simulink model "VHF_central_unit"  (R2024a)
settings: Solver=FixedStepDiscrete  StartTime=0.0  StopTime=10.0  FixedStep=0.001  RelTol=1e-3  EnableMultiTasking=on
PreLoadFcn:
  | try
  | MDL_install;
  | catch
  | end
InitFcn:
  | EcoCoder_PreCheckLic();
undefined symbols (not defined in the file or in its folder): C_ROTSPD_ZERO, C_SOC_ZERO, h, km, s, V
libraries: CoderSF_BSW_Libs x222, SF_CanService_Libs x16, CoderSF_ADC2Volt_Libs x6, CoderSF_6AxisMEMS_Libs x6, canmsglib x3, EV_ASWLibs x2, simulink x2, Chassis_stability_controllers x1, CoderSF_KeyCycle_Libs x1
(part 1 of 4)
CloseFcn:
  | try
  | MDL_uninstall;
  | catch
  | end
settings Model: Param_HCUVersion=EV22297A  Creator=HXL  LastModifiedBy=Henrique Mesquita
settings SolverCC: AlgebraicLoopSolver=TrustRegion
settings DataIOCC: ExternalInput=InputData  SaveFormat=Structure  SignalLoggingSaveFormat=ModelDataLogs  SaveOutput=off  SignalLogging=off  DSMLogging=off  SaveTime=off  ReturnWorkspaceOutputs=off
settings OptimizationCC: DefaultParameterBehavior=Inlined  InlineInvariantSignals=on  EnhancedBackFolding=on  StrengthReduction=on  EnableMemcpy=off  PassReuseOutputArgsAs=Individual arguments  ExpressionDepthLimit=2147483647  EfficientFloat2IntCast=on  LifeSpan=1  SimCompilerOptimization=on  OptimizeBlockOrder=speed  DifferentSizesBufferReuse=on  EfficientTunableParamExpr=on
settings DebuggingCC: AlgebraicLoopMsg=none  ArtificialAlgebraicLoopMsg=none  SaveWithDisabledLinksMsg=none  SaveWithParameterizedLinksMsg=none  CheckSSInitialOutputMsg=off  UnderspecifiedInitializationDetection=Classic  MergeDetectMultiDrivingBlocksExec=none  SignalResolutionControl=TryResolveAll  BlockPriorityViolationMsg=error  MinStepSizeMsg=none  InheritedTsInSrcMsg=none  MultiTaskDSMMsg=none  MultiTaskCondExecSysMsg=none  MultiTaskRateTransMsg=warning  TasksWithSamePriorityMsg=none  SigSpecEnsureSampleTimeMsg=none  IntegerOverflowMsg=error  Int32ToFloatConvMsg=none  ParameterPrecisionLossMsg=none  ParameterTunabilityLossMsg=none  FixptConstOverflowMsg=error  FcnCallInpInsideContextMsg=warning  UnconnectedInputMsg=error  UnconnectedOutputMsg=error  UnconnectedLineMsg=error  FrameProcessingCompatibilityMsg=none  BusObjectLabelMismatch=none  RootOutportRequireBusObject=none  UnknownTsInhSupMsg=none  ModelReferenceDataLoggingMessage=none  OperatingPointInterfaceChecksumMismatchMsg=none  SFUnusedDataAndEventsDiag=none  SFUnexpectedBacktrackingDiag=none  SFInvalidInputDataAccessInChartInitDiag=none  SFNoUnconditionalDefaultTransitionDiag=none  SFTransitionOutsideNaturalParentDiag=none  SFUnreachableExecutionPathDiag=none  SFExecutionAtInitializationDiag=none  IntegerSaturationMsg=error  ArithmeticOperatorsInVariantConditions=warning
settings HardwareCC: ProdBitPerPointer=32  ProdBitPerSizeT=32  ProdBitPerPtrDiffT=32  ProdLargestAtomicFloat=None  ProdWordSize=32  ProdHWDeviceType=Infineon->TriCore  TargetIntDivRoundTo=Zero  TargetEndianess=BigEndian  TargetHWDeviceType=Freescale->MPC55xx
settings ModelReferenceCC: UpdateModelReferenceTargets=Force  ModelReferenceNumInstancesAllowed=Single  PropagateSignalLabelsOutOfModel=off
settings SFSimCC: SFSimEcho=off  SimUseLocalCustomCode=off  MATLABDynamicMemAlloc=off  CustomCodeUndefinedFunction=UseInterfaceOnly
settings RTWCC: Description=Ecotrons TC2xx  SystemTargetFile=EcoCoderTC27x.tlc  GenerateMakefile=off  TemplateMakefile=ert_default_tmf  RTWVerbose=off  RetainRTWFile=on  RTWUseLocalCustomCode=off  RTWCompilerOptimization=on  GPUComputeCapability=3.5
settings CodeAppCC: IgnoreCustomStorageClasses=off  OperatorAnnotations=on  CustomSymbolStrGlobalVar=$N$M  CustomSymbolStrType=$N$M  CustomSymbolStrFcn=$N$M  CustomSymbolStrFcnArg=$N$M  CustomSymbolStrBlkIO=$N$M  CustomSymbolStrMacro=$N$M  InternalIdentifier=Classic
settings STFCustomTargetCC: TargetLangStandard=C89/C90 (ANSI)  CodeReplacementLibrary=ANSI_C  UtilityFuncGeneration=Shared location  MultiwordLength=256  IncludeMdlTerminateFcn=off  CombineOutputUpdateFcns=on  SuppressErrorStatus=on  ERTCustomFileBanners=on  SupportNonFinite=off  SupportComplex=off  SupportContinuousTime=off  SupportNonInlinedSFcns=off  MATLABClassNameForMDSCustomization=Simulink.SoftwareTarget.ERTCustomization  GRTInterface=off  UseToolchainInfoCompliant=off  SystemTargetFile=EcoCoderTC27x.tlc
settings ERTTargetCC: CodeReplacementLibrary=ANSI_C  UtilityFuncGeneration=Shared location  ParMdlRefBuildCompliant=off  CompOptLevelCompliant=off  ConcurrentExecutionCompliant=off  IncludeMdlTerminateFcn=off  SuppressErrorStatus=on  SupportNonFinite=off  SupportComplex=off  RemoveResetFunc=off  ModelStepFunctionPrototypeControlCompliant=off  CPPClassGenCompliant=off  UseToolchainInfoCompliant=off  GenerateASAP2=on  InlinedParameterPlacement=NonHierarchical  ERTCustomFileTemplate=MPC5644A_file_process.tlc  ERTFilePackagingFormat=Compact  PreserveIfCondition=on  ConvertIfToSwitch=off  PreserveExternInFcnDecls=off  SuppressUnreachableDefaultCases=off
settings ConfigComp: CovMetricSettings=dw  CovSaveCumulativeToWorkspaceVar=on  CovSaveSingleToWorkspaceVar=on  CovExternalEMLEnable=off  DVMaxProcessTime=3600  DVModelCoverageObjectives=MCDC  DVMaxTestCaseSteps=500  DVTestSuiteOptimization=CombinedObjectives  DVDetectActiveLogic=on  DVHarnessSource=Signal Editor

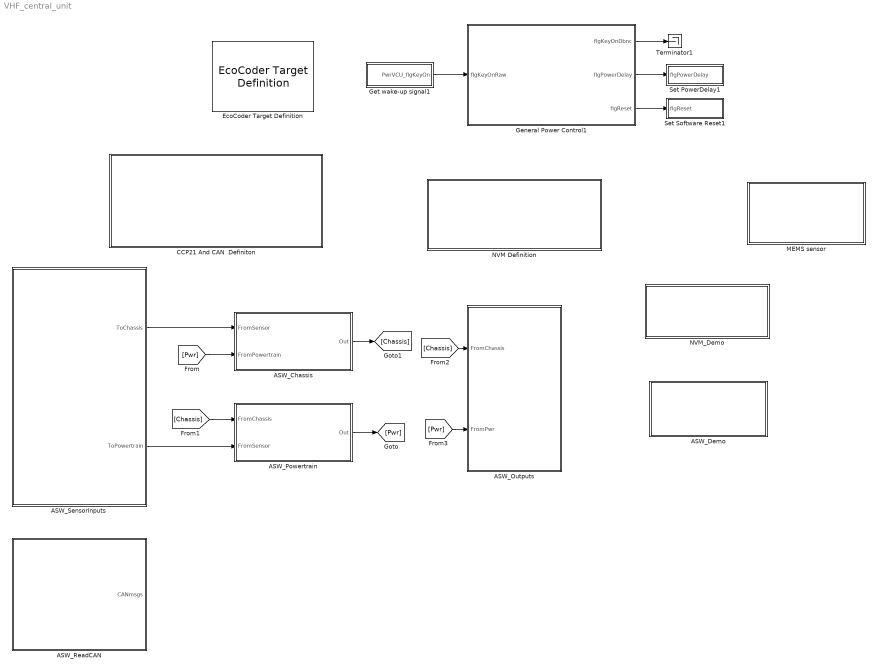
== system VHF_central_unit ==
  ASW_Chassis : Subsystem
  ASW_Demo : Subsystem  Priority=3
      settings: AttributesFormatString=%<Priority>
  ASW_Outputs : Subsystem
  ASW_Powertrain : Subsystem
  ASW_ReadCAN : Subsystem
  ASW_SensorInputs : Subsystem
  CCP21 And CAN  Definiton : Subsystem
  EcoCoder Target Definition : CoderSF_BSW_Libs/EcoCoder Target Definition  targetECU=EV22297A  EcoCoderBlockID=T001_Target  enNoTriggerCall=on  flgBlockReduction=on  flgShowDebugDisp=off  flgDisTargetOutFIleCounter=off  flgClearAllOldFiles=on  tc275_cal_len=hex2dec('00008000')  ipVal='192.168.0.123'  userName='nvidia'  passWord='nvidia'  workSpace='~/cmake_ws'  libraryLink=''  enExt=on  portExt=17725  Thread_D_pers=[1,1,5,10,20]  Thread_D_sizesStackDW=[500,380,350,360,370]  Thread_D_prioritysVal=[23,9,16,17,18]  internal_flash=[hex2dec('00020000'),hex2dec('000E0000')]  cal_rom_phy=[hex2dec('00010000'),hex2dec('00002000')]  cal_ram_wp=[hex2dec('4000F000'),hex2dec('00002000')]  cal_ram_msm=[hex2dec('40000000'),hex2dec('00002000')]  var_ram_wp=[hex2dec('40002000'),hex2dec('0000D000')]  write_back_fixed_ram=[hex2dec('40011000'),hex2dec('00001000')]  write_back_unfixed_ram=[hex2dec('40012000'),hex2dec('00001000')]  stack=[hex2dec('40013000'),hex2dec('00001000')]
      settings: AttributesFormatString=Target :%<targetECU>
  General Power Control1 : Subsystem  Priority=1  TreatAsAtomicUnit=on  mask(General Power Control V1.2){}
      settings: AttributesFormatString=Priority:%<Priority>
      mask Display: disp('Power Control V2.0');
  Get wake-up signal1 : Subsystem
  MEMS sensor : Subsystem
  NVM Definition : Subsystem
  NVM_Demo : Subsystem  Priority=2
      settings: AttributesFormatString=%<Priority>
  Set PowerDelay1 : Subsystem
  Set Software Reset1 : Subsystem
  Terminator1 : Terminator
  wires:
  General Power Control1/1(flgKeyOnDbnc) -> Terminator1/1
  General Power Control1/3(flgReset) -> Set Software Reset1/1(flgReset)
  Get wake-up signal1/1(PwrVCU_flgKeyOn) -> General Power Control1/1(flgKeyOnRaw)
  General Power Control1/2(flgPowerDelay) -> Set PowerDelay1/1(flgPowerDelay)
  ASW_SensorInputs/2(ToPowertrain) -> ASW_Powertrain/2(FromSensor)
  ASW_SensorInputs/1(ToChassis) -> ASW_Chassis/1(FromSensor)
  [Pwr] -> ASW_Chassis/2(FromPowertrain)
  [Chassis] -> ASW_Powertrain/1(FromChassis)
  ASW_Chassis/1(Out) -> [Chassis]
  ASW_Powertrain/1(Out) -> [Pwr]
  [Chassis] -> ASW_Outputs/1(FromChassis)
  [Pwr] -> ASW_Outputs/2(FromPwr)

== system VHF_central_unit/ASW_Chassis ==
  FromSensor : Inport
  FromPowertrain : Inport  Port=2
  Electronic Differential control : Subsystem
  Reasoning : Subsystem
  Vehicle Longitudinal Control : Subsystem
  Out : Outport

== system VHF_central_unit/ASW_Demo ==
  01  process input signals : Subsystem
  02 vehicle motion request : Subsystem
  03 electrical supply management : Subsystem
  "04 powertrain control " : Subsystem
  05 thermal management : Subsystem
  06 process output signals : Subsystem
  wires:
  01  process input signals/4(sigInTm_rotspd) -> "04 powertrain control "/3(sigInTm_rotspd)
  05 thermal management/1(thrmlFan_flgCoolLoSpdEn) -> 06 process output signals/4(thrmlFan_flgCoolLoSpdEn)
  "04 powertrain control "/2(pwrtrnBmscPack_flgConnReq) -> 06 process output signals/3(pwrtrnBmscPack_flgConnReq)
  "04 powertrain control "/1(pwrtrnTmc_trqCmd) -> 06 process output signals/2(pwrtrnTmc_trqCmd)
  03 electrical supply management/1(esmcDcdc_flgEn) -> 06 process output signals/1(esmcDcdc_flgEn)
  01  process input signals/3(sigInBms_soc) -> "04 powertrain control "/2(sigInBms_soc)
  02 vehicle motion request/1(vehDrv_trqReq) -> "04 powertrain control "/1(vehDrv_trqReq)
  01  process input signals/2(sigInDrvPedacc_pct) -> 02 vehicle motion request/1(sigInDrvPedacc_pct)
  01  process input signals/1(sigInEsmBatt_volt) -> 03 electrical supply management/1(sigInEsmBatt_volt)

== system VHF_central_unit/ASW_Outputs ==
  FromChassis : Inport
  FromPwr : Inport  Port=2
  Command DCDC Converter : Subsystem
  Command GenSys : Subsystem
  Command Inverter 1 : Subsystem
  Command Inverter 2 : Subsystem

== system VHF_central_unit/ASW_Powertrain ==
  FromChassis : Inport
  FromSensor : Inport  Port=2
  Command DCDC Converter : Subsystem
  Command GenSys : Subsystem
  Command Inverter 1 : Subsystem
  Command Inverter 2 : Subsystem
  Energy management : Subsystem
  System Protection : Subsystem
  Out : Outport

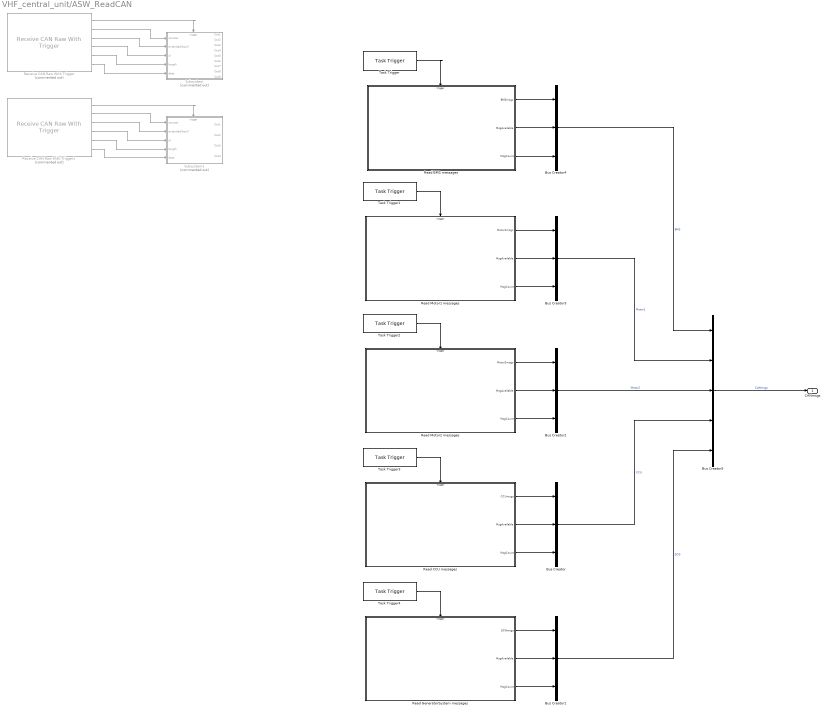
== system VHF_central_unit/ASW_ReadCAN ==
  Bus Creator{,1..4} (5 alike) : BusCreator  Inputs=3
  Bus Creator5 : BusCreator  Inputs=5
  Read BMS messages : Subsystem
  Read CCU messages : Subsystem
  Read GeneratorSystem messages : Subsystem
  Read Motor1 messages : Subsystem
  Read Motor2 messages : Subsystem
  Receive CAN Raw With Trigger : CoderSF_BSW_Libs/CAN/Receive CAN Raw With Trigger  Commented=on  channel=CAN_A
  Receive CAN Raw With Trigger1 : CoderSF_BSW_Libs/CAN/Receive CAN Raw With Trigger  Commented=on  channel=CAN_B
  Subsystem : Subsystem  Commented=on
  Subsystem1 : Subsystem  Commented=on
  Task Trigger{,1..4} (5 alike) : CoderSF_BSW_Libs/Task Scheduler/Task Trigger  tasktimeIndex=Task_L20ms
  CANmsgs : Outport
  wires:
  Receive CAN Raw With Trigger/2 -> Subsystem/1(remote)
  Receive CAN Raw With Trigger/3 -> Subsystem/2(extended(bool))
  Receive CAN Raw With Trigger/4 -> Subsystem/3(id)
  Receive CAN Raw With Trigger/5 -> Subsystem/4(length)
  Receive CAN Raw With Trigger/6 -> Subsystem/5(data)
  Receive CAN Raw With Trigger/1 -> Subsystem/Trigger
  Receive CAN Raw With Trigger1/4 -> Subsystem1/3(id)
  Receive CAN Raw With Trigger1/3 -> Subsystem1/2(extended(bool))
  Receive CAN Raw With Trigger1/6 -> Subsystem1/5(data)
  Receive CAN Raw With Trigger1/5 -> Subsystem1/4(length)
  Receive CAN Raw With Trigger1/2 -> Subsystem1/1(remote)
  Receive CAN Raw With Trigger1/1 -> Subsystem1/Trigger
  Task Trigger/1 -> Read BMS messages/Trigger
  Task Trigger3/1 -> Read CCU messages/Trigger
  Task Trigger4/1 -> Read GeneratorSystem messages/Trigger
  Task Trigger1/1 -> Read Motor1 messages/Trigger
  Task Trigger2/1 -> Read Motor2 messages/Trigger
  Read CCU messages/2(MsgAvailable) -> Bus Creator/2
  Read CCU messages/1(CCUmsgs) -> Bus Creator/1
  Read CCU messages/3(MsgCount) -> Bus Creator/3
  Read GeneratorSystem messages/1(SCGmsgs) -> Bus Creator1/1
  Read GeneratorSystem messages/2(MsgAvailable) -> Bus Creator1/2
  Read GeneratorSystem messages/3(MsgCount) -> Bus Creator1/3
  Read Motor2 messages/3(MsgCount) -> Bus Creator2/3
  Read Motor2 messages/2(MsgAvailable) -> Bus Creator2/2
  Read Motor2 messages/1(Motor2msgs) -> Bus Creator2/1
  Read Motor1 messages/1(Motor1msgs) -> Bus Creator3/1
  Read Motor1 messages/2(MsgAvailable) -> Bus Creator3/2
  Read Motor1 messages/3(MsgCount) -> Bus Creator3/3
  Read BMS messages/1(BMSmsgs) -> Bus Creator4/1
  Read BMS messages/2(MsgAvailable) -> Bus Creator4/2
  Read BMS messages/3(MsgCount) -> Bus Creator4/3
  Bus Creator5/1 -> CANmsgs/1  "CANmsgs"
  Bus Creator2/1 -> Bus Creator5/3  "Motor2"
  Bus Creator3/1 -> Bus Creator5/2  "Motor1"
  Bus Creator4/1 -> Bus Creator5/1  "BMS"
  Bus Creator/1 -> Bus Creator5/4  "CCU"
  Bus Creator1/1 -> Bus Creator5/5  "SCG"

== system VHF_central_unit/ASW_SensorInputs ==
  02 vehicle motion request : Subsystem
  Accelerator read : Subsystem
  Brake read : Subsystem
  MEMS sensor read : Subsystem
  Output Routing : Subsystem
  Read BMS msgs : Subsystem
  Read DCDC converter msgs : Subsystem
  Read GenSys msgs : Subsystem
  Read Inverter 1 : Subsystem
  Read Inverter 2 : Subsystem
  ToChassis : Outport
  ToPowertrain : Outport  Port=2
  wires:
  Accelerator read/1(thrtl) -> 02 vehicle motion request/1(sigInDrvPedacc_pct)
  Brake read/1(brk) -> ?
  Output Routing/2(ToPowertrain) -> ToPowertrain/1
  Output Routing/1(ToChassis) -> ToChassis/1

== system VHF_central_unit/CCP21 And CAN  Definiton ==
  CAN Channel Definition : CoderSF_BSW_Libs/CAN/CAN Channel Definition  channel=CAN_A  can_en=on  can_idfilter=off  can_rxextended=on  can_rxMask=hex2dec('0')  can_rxID=hex2dec('200')  can_baudrateIndex=500  can_txbuffer_size=hex2dec('60')  can_rxbuffer_size=1  can_en_fd=off  nominalSamplePoint=7500  can_baudrateIndex_data=1000  fastSamplePoint=7500  canfd_txbuffer_size=5  EcoCoderBlockID=C001_CANDef
  CAN Channel Definition1 : CoderSF_BSW_Libs/CAN/CAN Channel Definition  channel=CAN_B  can_en=on  can_idfilter=off  can_rxextended=on  can_rxMask=hex2dec('0')  can_rxID=hex2dec('800')  can_baudrateIndex=500  can_txbuffer_size=30  can_rxbuffer_size=1  can_en_fd=off  nominalSamplePoint=7500  can_baudrateIndex_data=1000  fastSamplePoint=7500  canfd_txbuffer_size=5  EcoCoderBlockID=C001_CANDef
  CAN Channel Definition2 : CoderSF_BSW_Libs/CAN/CAN Channel Definition  channel=CAN_C  can_en=on  can_idfilter=off  can_rxextended=on  can_rxMask=hex2dec('0')  can_rxID=hex2dec('100')  can_baudrateIndex=500  can_txbuffer_size=hex2dec('A')+hex2dec('20')+hex2dec('30')+hex2dec('50')+5  can_rxbuffer_size=1  can_en_fd=off  nominalSamplePoint=7500  can_baudrateIndex_data=1000  fastSamplePoint=7500  canfd_txbuffer_size=5  EcoCoderBlockID=C001_CANDef
  CAN Channel Definition3 : CoderSF_BSW_Libs/CAN/CAN Channel Definition  channel=CAN_D  can_en=on  can_idfilter=on  can_rxextended=on  can_rxMask=hex2dec('0')  can_rxID=hex2dec('100')  can_baudrateIndex=250  can_txbuffer_size=hex2dec('A')+hex2dec('20')+hex2dec('30')+hex2dec('50')+5  can_rxbuffer_size=1  can_en_fd=off  nominalSamplePoint=7500  can_baudrateIndex_data=1000  fastSamplePoint=7500  canfd_txbuffer_size=5  EcoCoderBlockID=C001_CANDef
  CAN Channel Definition4 : CoderSF_BSW_Libs/CAN/CAN Channel Definition  channel=CAN_E  can_en=on  can_idfilter=on  can_rxextended=on  can_rxMask=hex2dec('0')  can_rxID=hex2dec('100')  can_baudrateIndex=250  can_txbuffer_size=hex2dec('A')+hex2dec('20')+hex2dec('30')+hex2dec('50')+5  can_rxbuffer_size=1  can_en_fd=off  nominalSamplePoint=7500  can_baudrateIndex_data=1000  fastSamplePoint=7500  canfd_txbuffer_size=5  EcoCoderBlockID=C001_CANDef
  CAN Channel Definition5 : CoderSF_BSW_Libs/CAN/CAN Channel Definition  channel=CAN_F  can_en=on  can_idfilter=on  can_rxextended=on  can_rxMask=hex2dec('0')  can_rxID=hex2dec('100')  can_baudrateIndex=500  can_txbuffer_size=hex2dec('A')+hex2dec('20')+hex2dec('30')+hex2dec('50')+5  can_rxbuffer_size=1  can_en_fd=off  nominalSamplePoint=7500  can_baudrateIndex_data=1000  fastSamplePoint=7500  canfd_txbuffer_size=5  EcoCoderBlockID=C001_CANDef
  Fixed CCP Slave Definition : CoderSF_BSW_Libs/CCP/Fixed CCP Slave Definition  ccp_enSet=on  ccp_disASW=off  channel=CAN_C  stationaddressSet=hex2dec('0112')  croidSet=hex2dec('200')  dtoidSet=hex2dec('201')  daqidSet=[hex2dec('210') hex2dec('211') hex2dec('212') hex2dec('213')]  daqpidSet=[hex2dec('0') hex2dec('0') hex2dec('0') hex2dec('0')]  daqlenSet=[hex2dec('A') hex2dec('20') hex2dec('30') hex2dec('50')]  dtoTaskTrigger=Task_H1ms  daq0TaskTrigger=Task_L1ms  daq1TaskTrigger=Task_L1ms  daq2TaskTrigger=Task_L1ms  daq3TaskTrigger=Task_L1ms  daqperSet=[10 20 100 200]  EcoCoderBlockID=C002_CCP21Conf

== system VHF_central_unit/General Power Control1 ==
  flgKeyOnRaw : Inport
  Constant1 : Constant  Value=0
  Control KeyCycle : Subsystem
  Control Restore All NVM Data : Subsystem
  Debounce KeyOn : Subsystem
  Enable Restore And Store NVM : Subsystem
  Read Calibration2 : CoderSF_BSW_Libs/Calibration & Measurement/Read Calibration  variable_name=PwrMCU_flgEnRestoreStoreNVM_val  variable_value=0  variable_type=boolean  variable_min=[]  variable_max=[]  unitStr=""  descStr=""
      settings: AttributesFormatString=value:%<variable_value> type:%<variable_type> max:%<variable_max> Min:%<variable_min>
  Shut Down MCU : Subsystem
  Task Trigger1 : CoderSF_BSW_Libs/Task Scheduler/Task Trigger  tasktimeIndex=Task_ini
  Task Trigger{2..5} (4 alike) : CoderSF_BSW_Libs/Task Scheduler/Task Trigger  tasktimeIndex=Task_L5ms
  flgKeyOnDbnc : Outport
  flgPowerDelay : Outport  Port=2
  flgReset : Outport  Port=3
  wires:
  Constant1/1 -> Shut Down MCU/1(flgForcePwrOffMCU)
  Shut Down MCU/1(flgPowerDelay) -> flgPowerDelay/1
  Task Trigger2/1 -> Control KeyCycle/Trigger
  flgKeyOnRaw/1 -> Debounce KeyOn/1(flgKeyOnRaw)
  Task Trigger3/1 -> Debounce KeyOn/Trigger
  Task Trigger4/1 -> Shut Down MCU/Trigger
  Task Trigger1/1 -> Control Restore All NVM Data/Trigger
  Control KeyCycle/1(flgReset) -> flgReset/1
  Debounce KeyOn/1(PwrMCU_flgKeyOnDbnc) -> Control KeyCycle/1(flgKeyon_raw), flgKeyOnDbnc/1, Enable Restore And Store NVM/1(flgKeyon), Shut Down MCU/2(flgKeyon)
  Enable Restore And Store NVM/1(flgEnStoreNVM) -> Shut Down MCU/3(flgEnNVMStore)
  Task Trigger5/1 -> Enable Restore And Store NVM/Trigger
  Read Calibration2/1 -> Enable Restore And Store NVM/2(flgEnRestoreStoreNVM_val), Control Restore All NVM Data/1(flgEnNVMRestore)

== system VHF_central_unit/Get wake-up signal1 ==
  Get wake-up signal : Subsystem
  Task Trigger3 : CoderSF_BSW_Libs/Task Scheduler/Task Trigger  tasktimeIndex=Task_L5ms
  Write and Read Measurement1 : CoderSF_BSW_Libs/Calibration & Measurement/Write and Read Measurement  variable_name=PwrMCU_flgKeyOnRaw  variable_value=0  variable_type=boolean  numD=1  unitStr=""  descStr=""
      settings: AttributesFormatString=type:%<variable_type> Dimensions:%<numD>
  PwrVCU_flgKeyOn : Outport
  wires:
  Task Trigger3/1 -> Get wake-up signal/Trigger
  Get wake-up signal/1(PwrVCU_flgKeyOn) -> Write and Read Measurement1/1
  Write and Read Measurement1/1 -> PwrVCU_flgKeyOn/1  "PwrMCU_flgKeyOnRaw"

== system VHF_central_unit/MEMS sensor ==
  6-Axis MEMS Sensor Definition : CoderSF_6AxisMEMS_Libs/6-Axis MEMS Sensor/6-Axis MEMS Sensor Definition  gyro_fs=250  accel_fs=2  gyro_bw=176  accel_bw=218
  Sensor Self Test : Subsystem
  Task Trigger : CoderSF_BSW_Libs/Task Scheduler/Task Trigger  Priority=6  tasktimeIndex=Task_ini  PrioritySet=6
  wires:
  Task Trigger/1 -> Sensor Self Test/Trigger

== system VHF_central_unit/NVM Definition ==
  Fixed NVM Definition : CoderSF_BSW_Libs/Non-volatile Memory Blocks/Fixed NVM Definition  EcoCoderBlockID=F001_FNVMDef  nvmDefData=vcu_getFixedNvmList

== system VHF_central_unit/NVM_Demo ==
  NVM_Read : Subsystem
  NVM_ReadAndWrite : Subsystem
  Task_Call1 : CoderSF_BSW_Libs/Task Scheduler/Task Trigger  tasktimeIndex=Task_L20ms
  Task_Call2 : CoderSF_BSW_Libs/Task Scheduler/Task Trigger  tasktimeIndex=Task_ini
  wires:
  Task_Call2/1 -> NVM_ReadAndWrite/Trigger
  Task_Call1/1 -> NVM_Read/Trigger

== system VHF_central_unit/Set PowerDelay1 ==
  flgPowerDelay : Inport
  "Set PowerDelay of Switch Internal " : Subsystem
  Task_Trigger : CoderSF_BSW_Libs/Task Scheduler/Task Trigger  tasktimeIndex=Task_L5ms
  wires:
  flgPowerDelay/1 -> "Set PowerDelay of Switch Internal "/1(flgPowerDelay)
  Task_Trigger/1 -> "Set PowerDelay of Switch Internal "/Trigger

== system VHF_central_unit/Set Software Reset1 ==
  flgReset : Inport
  Set Software Reset : Subsystem
  Task_Trigger : CoderSF_BSW_Libs/Task Scheduler/Task Trigger  tasktimeIndex=Task_L5ms
  wires:
  Task_Trigger/1 -> Set Software Reset/Trigger
  flgReset/1 -> Set Software Reset/1(flgReset)

== system VHF_central_unit/ASW_Chassis/Electronic Differential control ==
  thrtl : Inport
  brk : Inport  Port=2
  Constant : Constant
  Terminator : Terminator
  Terminator1 : Terminator
  Out1 : Outport
  wires:
  thrtl/1 -> Terminator/1
  brk/1 -> Terminator1/1
  Constant/1 -> Out1/1

== system VHF_central_unit/ASW_Chassis/Reasoning ==
  thrtl : Inport
  brk : Inport  Port=2
  Constant : Constant
  Terminator : Terminator
  Terminator1 : Terminator
  Out1 : Outport
  wires:
  thrtl/1 -> Terminator/1
  brk/1 -> Terminator1/1
  Constant/1 -> Out1/1

== system VHF_central_unit/ASW_Chassis/Vehicle Longitudinal Control ==
  thrtl : Inport
  brk : Inport  Port=2
  Constant : Constant
  Terminator : Terminator
  Terminator1 : Terminator
  TractionController : Chassis_stability_controllers/TractionController  SystemSampleTime=-1  VariantActivationTime=update diagram  AllowFlexibleInterface=on  Latency=0  AutoFrameSizeCalculation=off
  Out1 : Outport
  wires:
  thrtl/1 -> Terminator/1
  brk/1 -> Terminator1/1
  Constant/1 -> Out1/1

== system VHF_central_unit/ASW_Demo/01  process input signals ==
  01 process electrical supply input signals : Subsystem
  02 process driver input signals : Subsystem
  03 process bms input signals : Subsystem
  04 process traction motor input signals : Subsystem
  sigInEsmBatt_volt : Outport
  sigInDrvPedacc_pct : Outport  Port=2
  sigInBms_soc : Outport  Port=3
  sigInTm_rotspd : Outport  Port=4
  wires:
  04 process traction motor input signals/1(sigInTm_rotspd) -> sigInTm_rotspd/1
  02 process driver input signals/1(sigInDrvPedacc_pct) -> sigInDrvPedacc_pct/1
  01 process electrical supply input signals/1(sigInEsmBatt_volt) -> sigInEsmBatt_volt/1
  03 process bms input signals/1(sigInBms_soc) -> sigInBms_soc/1

== system VHF_central_unit/ASW_Demo/02 vehicle motion request ==
  sigInDrvPedacc_pct : Inport
  01 driver torque demand : Subsystem
  Task_Call2 : CoderSF_BSW_Libs/Task Scheduler/Task Trigger  tasktimeIndex=Task_L20ms
  vehDrv_trqReq : Outport
  wires:
  Task_Call2/1 -> 01 driver torque demand/Trigger
  01 driver torque demand/1(vehDrv_trqReq1) -> vehDrv_trqReq/1
  sigInDrvPedacc_pct/1 -> 01 driver torque demand/1(sigInDrvPedacc_pct1)

== system VHF_central_unit/ASW_Demo/03 electrical supply management ==
  sigInEsmBatt_volt : Inport
  02  electrical supply control : Subsystem
  esmcDcdc_flgEn : Outport
  wires:
  02  electrical supply control/1(esmcDcdc_flgEn) -> esmcDcdc_flgEn/1
  sigInEsmBatt_volt/1 -> 02  electrical supply control/1(sigInEsmBatt_volt)

== system VHF_central_unit/ASW_Demo/04 powertrain control  ==
  vehDrv_trqReq : Inport
  sigInBms_soc : Inport  Port=2
  sigInTm_rotspd : Inport  Port=3
  02  Bms control : Subsystem
  03  traction motor control : Subsystem
  pwrtrnTmc_trqCmd : Outport
  pwrtrnBmscPack_flgConnReq : Outport  Port=2
  wires:
  02  Bms control/1(pwrtrnBmscPack_flgConnReq) -> pwrtrnBmscPack_flgConnReq/1
  03  traction motor control/1(pwrtrnTmc_trqCmd) -> pwrtrnTmc_trqCmd/1
  sigInTm_rotspd/1 -> 03  traction motor control/1(sigInTm_rotspd)
  sigInBms_soc/1 -> 02  Bms control/1(sigInBms_soc)
  vehDrv_trqReq/1 -> 03  traction motor control/2(vehDrv_trqReq)

== system VHF_central_unit/ASW_Demo/05 thermal management ==
  Task_Call4 : CoderSF_BSW_Libs/Task Scheduler/Task Trigger  tasktimeIndex=Task_L100ms
  thrml : Subsystem
  thrmlFan_flgCoolLoSpdEn : Outport
  wires:
  Task_Call4/1 -> thrml/Trigger
  thrml/1(thrmlFan_flgCoolLoSpdEn) -> thrmlFan_flgCoolLoSpdEn/1

== system VHF_central_unit/ASW_Demo/06 process output signals ==
  esmcDcdc_flgEn : Inport
  pwrtrnTmc_trqCmd : Inport  Port=2
  pwrtrnBmscPack_flgConnReq : Inport  Port=3
  thrmlFan_flgCoolLoSpdEn : Inport  Port=4
  01 process electrical supply output signals : Subsystem
  02 process traction motor output signals : Subsystem
  03 process bms output signals : Subsystem
  Terminator1 : Terminator
  wires:
  pwrtrnTmc_trqCmd/1 -> 02 process traction motor output signals/1(pwrtrnTmc_trqCmd)
  esmcDcdc_flgEn/1 -> 01 process electrical supply output signals/1(esmcDcdc_flgEn)
  pwrtrnBmscPack_flgConnReq/1 -> 03 process bms output signals/1(pwrtrnBmscPack_flgConnReq)
  thrmlFan_flgCoolLoSpdEn/1 -> Terminator1/1

== system VHF_central_unit/ASW_Outputs/Command DCDC Converter ==
  In1 : Inport
  Subsystem1 : Subsystem
  Task Trigger : CoderSF_BSW_Libs/Task Scheduler/Task Trigger  tasktimeIndex=Task_L20ms
  wires:
  Task Trigger/1 -> Subsystem1/Trigger
  In1/1 -> Subsystem1/1(In1)

== system VHF_central_unit/ASW_Outputs/Command GenSys ==
  In1 : Inport
  Subsystem1 : Subsystem
  Task Trigger : CoderSF_BSW_Libs/Task Scheduler/Task Trigger  tasktimeIndex=Task_L20ms
  wires:
  Task Trigger/1 -> Subsystem1/Trigger
  In1/1 -> Subsystem1/1(In1)

== system VHF_central_unit/ASW_Outputs/Command Inverter 1 ==
  In1 : Inport
  Subsystem1 : Subsystem
  Task Trigger : CoderSF_BSW_Libs/Task Scheduler/Task Trigger  tasktimeIndex=Task_L20ms
  wires:
  Task Trigger/1 -> Subsystem1/Trigger
  In1/1 -> Subsystem1/1(In1)

== system VHF_central_unit/ASW_Outputs/Command Inverter 2 ==
  In1 : Inport
  Subsystem1 : Subsystem
  Task Trigger : CoderSF_BSW_Libs/Task Scheduler/Task Trigger  tasktimeIndex=Task_L20ms
  wires:
  Task Trigger/1 -> Subsystem1/Trigger
  In1/1 -> Subsystem1/1(In1)

== system VHF_central_unit/ASW_Powertrain/Command DCDC Converter ==
  In1 : Inport
  Subsystem1 : Subsystem
  Task Trigger : CoderSF_BSW_Libs/Task Scheduler/Task Trigger  tasktimeIndex=Task_L20ms
  wires:
  Task Trigger/1 -> Subsystem1/Trigger
  In1/1 -> Subsystem1/1(In1)

== system VHF_central_unit/ASW_Powertrain/Command GenSys ==
  In1 : Inport
  Subsystem1 : Subsystem
  Task Trigger : CoderSF_BSW_Libs/Task Scheduler/Task Trigger  tasktimeIndex=Task_L20ms
  wires:
  Task Trigger/1 -> Subsystem1/Trigger
  In1/1 -> Subsystem1/1(In1)

== system VHF_central_unit/ASW_Powertrain/Command Inverter 1 ==
  In1 : Inport
  Subsystem1 : Subsystem
  Task Trigger : CoderSF_BSW_Libs/Task Scheduler/Task Trigger  tasktimeIndex=Task_L20ms
  wires:
  Task Trigger/1 -> Subsystem1/Trigger
  In1/1 -> Subsystem1/1(In1)

== system VHF_central_unit/ASW_Powertrain/Command Inverter 2 ==
  In1 : Inport
  Subsystem1 : Subsystem
  Task Trigger : CoderSF_BSW_Libs/Task Scheduler/Task Trigger  tasktimeIndex=Task_L20ms
  wires:
  Task Trigger/1 -> Subsystem1/Trigger
  In1/1 -> Subsystem1/1(In1)

== system VHF_central_unit/ASW_Powertrain/Energy management ==
  In1 : Inport
  Out1 : Outport
  wires:
  In1/1 -> Out1/1

== system VHF_central_unit/ASW_Powertrain/System Protection ==
  In1 : Inport
  Out1 : Outport
  wires:
  In1/1 -> Out1/1

== system VHF_central_unit/ASW_ReadCAN/Read BMS messages ==
  function : TriggerPort  TriggerType=function-call  VariantControl=(inherit)
  Bus Creator : BusCreator  Inputs=4
  Bus Creator1 : BusCreator  Inputs=7
  Bus Creator2 : BusCreator  Inputs=10
  Bus Creator3 : BusCreator  Inputs=7
  Bus Creator4 : BusCreator  Inputs=10
  Read CAN Message : SF_CanService_Libs/Read CAN Message  typeCAN=Connected  channel=CAN_A  mEn=off  msgInfo=VHF_VCU_Msg  msgItermStore=BMS_CellVoltage1to8  msgIterm=BMS_CellVoltage1to8  valid=on  stale=on  motoBit=off  setSignalName=on  flgCustomMonitorVariableRules=off  defineSignalName=on  prefixSignal='BMS'  flgValTest=off  flgNoFixed=on  flgInheritForNoFixed=off  tSample=Task_Inherit  modeCode=Parameterized
  Read CAN Message1 : SF_CanService_Libs/Read CAN Message  typeCAN=Connected  channel=CAN_A  mEn=off  msgInfo=VHF_VCU_Msg  msgItermStore=BMS_CellVoltage9to16  msgIterm=BMS_CellVoltage9to16  valid=on  stale=on  motoBit=off  setSignalName=on  flgCustomMonitorVariableRules=off  defineSignalName=on  prefixSignal='BMS'  flgValTest=off  flgNoFixed=on  flgInheritForNoFixed=off  tSample=Task_Inherit  modeCode=Parameterless
  Read CAN Message2 : SF_CanService_Libs/Read CAN Message  typeCAN=Connected  channel=CAN_A  mEn=off  msgInfo=VHF_VCU_Msg  msgItermStore=BMS_OperationStatus  msgIterm=BMS_OperationStatus  valid=on  stale=on  motoBit=off  setSignalName=on  flgCustomMonitorVariableRules=off  defineSignalName=on  prefixSignal='BMS'  flgValTest=off  flgNoFixed=on  flgInheritForNoFixed=off  tSample=Task_Inherit  modeCode=Parameterless
  Read CAN Message3 : SF_CanService_Libs/Read CAN Message  typeCAN=Connected  channel=CAN_A  mEn=off  msgInfo=VHF_VCU_Msg  msgItermStore=BMS_StateOfStatus  msgIterm=BMS_StateOfStatus  valid=on  stale=on  motoBit=off  setSignalName=on  flgCustomMonitorVariableRules=off  defineSignalName=on  prefixSignal='BMS'  flgValTest=off  flgNoFixed=on  flgInheritForNoFixed=off  tSample=Task_Inherit  modeCode=Parameterless
  Subsystem : Subsystem
  BMSmsgs : Outport
  MsgAvailable : Outport  Port=2
  MsgCount : Outport  Port=3
  wires:
  Read CAN Message2/3 -> Bus Creator1/3  "BMSBattPackVoltage"
  Read CAN Message2/4 -> Bus Creator1/4  "BMSBattOCV"
  Read CAN Message2/6 -> Bus Creator1/6  "BMSPackMaxDischargeCurrent"
  Read CAN Message2/5 -> Bus Creator1/5  "BMSBattPackCurrent"
  Read CAN Message2/7 -> Bus Creator1/7  "BMSPackMaxChargeCurrent"
  Read CAN Message3/4 -> Bus Creator3/4  "BMSStateOfHealth"
  Read CAN Message3/3 -> Bus Creator3/3  "BMSStateOfCharge"
  Read CAN Message3/5 -> Bus Creator3/5  "BMSStateOfEnergy"
  Read CAN Message3/6 -> Bus Creator3/6  "BMSBattStoragedEnergy"
  Read CAN Message3/7 -> Bus Creator3/7  "BMSBattTemperature"
  Read CAN Message2/2 -> Bus Creator1/2
  Read CAN Message2/1 -> Bus Creator1/1
  Read CAN Message3/1 -> Bus Creator3/1
  Read CAN Message3/2 -> Bus Creator3/2
  Read CAN Message/1 -> Bus Creator2/1
  Read CAN Message/2 -> Bus Creator2/2
  Read CAN Message/3 -> Bus Creator2/3  "BMSCellVoltage1"
  Read CAN Message/4 -> Bus Creator2/4  "BMSCellVoltage2"
  Read CAN Message/5 -> Bus Creator2/5  "BMSCellVoltage3"
  Read CAN Message/6 -> Bus Creator2/6  "BMSCellVoltage4"
  Read CAN Message/7 -> Bus Creator2/7  "BMSCellVoltage5"
  Read CAN Message/8 -> Bus Creator2/8  "BMSCellVoltage6"
  Read CAN Message/9 -> Bus Creator2/9  "BMSCellVoltage7"
  Read CAN Message/10 -> Bus Creator2/10  "BMSCellVoltage8"
  Read CAN Message1/10 -> Bus Creator4/10  "BMSCellVoltage16"
  Read CAN Message1/9 -> Bus Creator4/9  "BMSCellVoltage15"
  Read CAN Message1/8 -> Bus Creator4/8  "BMSCellVoltage14"
  Read CAN Message1/7 -> Bus Creator4/7  "BMSCellVoltage13"
  Read CAN Message1/6 -> Bus Creator4/6  "BMSCellVoltage12"
  Read CAN Message1/5 -> Bus Creator4/5  "BMSCellVoltage11"
  Read CAN Message1/4 -> Bus Creator4/4  "BMSCellVoltage10"
  Read CAN Message1/3 -> Bus Creator4/3  "BMSCellVoltage9"
  Read CAN Message1/2 -> Bus Creator4/2
  Read CAN Message1/1 -> Bus Creator4/1
  Bus Creator1/1 -> Bus Creator/1  "BMS_OperationStatus"
  Bus Creator3/1 -> Bus Creator/2  "BMS_StateOfStatus"
  Bus Creator2/1 -> Bus Creator/3  "BMS_CellVoltage1to8"
  Bus Creator4/1 -> Bus Creator/4  "BMS_CellVoltage9to16"
  Bus Creator/1 -> Subsystem/1(In1)
  Subsystem/2(MsgAvailable) -> MsgAvailable/1
  Subsystem/1(BMSmsgs) -> BMSmsgs/1
  Subsystem/3(MsgCount) -> MsgCount/1

== system VHF_central_unit/ASW_ReadCAN/Read CCU messages ==
  function : TriggerPort  TriggerType=function-call  VariantControl=(inherit)
  Bus Creator : BusCreator  Inputs=2
  Bus Creator1 : BusCreator  Inputs=17
  Bus Creator3 : BusCreator  Inputs=5
  Read CAN Message2 : SF_CanService_Libs/Read CAN Message  typeCAN=Connected  channel=CAN_A  mEn=off  msgInfo=VHF_VCU_Msg  msgItermStore=CCU_Status_VCU  msgIterm=CCU_Status_VCU  valid=on  stale=on  motoBit=off  setSignalName=on  flgCustomMonitorVariableRules=off  defineSignalName=on  prefixSignal='CCU'  flgValTest=off  flgNoFixed=on  flgInheritForNoFixed=off  tSample=Task_Inherit  modeCode=Parameterless
  Read CAN Message3 : SF_CanService_Libs/Read CAN Message  typeCAN=Connected  channel=CAN_A  mEn=off  msgInfo=VHF_VCU_Msg  msgItermStore=CCU_InductorStatus  msgIterm=CCU_InductorStatus  valid=on  stale=on  motoBit=off  setSignalName=on  flgCustomMonitorVariableRules=off  defineSignalName=on  prefixSignal='CCU'  flgValTest=off  flgNoFixed=on  flgInheritForNoFixed=off  tSample=Task_Inherit  modeCode=Parameterless
  Subsystem : Subsystem
  CCUmsgs : Outport
  MsgAvailable : Outport  Port=2
  MsgCount : Outport  Port=3
  wires:
  Read CAN Message2/8 -> Bus Creator1/8  "CCUFaultControl"
  Read CAN Message3/1 -> Bus Creator3/1
  Bus Creator3/1 -> Bus Creator/2  "CCU_InductorStatus"
  Read CAN Message3/3 -> Bus Creator3/3  "CCUInductor1Curr"
  Subsystem/1(CCUmsgs) -> CCUmsgs/1
  Read CAN Message3/4 -> Bus Creator3/4  "CCUInductor2Curr"
  Read CAN Message3/2 -> Bus Creator3/2
  Read CAN Message2/2 -> Bus Creator1/2
  Subsystem/3(MsgCount) -> MsgCount/1
  Read CAN Message2/5 -> Bus Creator1/5  "CCUInputCurrent"
  Bus Creator1/1 -> Bus Creator/1  "CCU_Status_VCU"
  Read CAN Message2/4 -> Bus Creator1/4  "CCUDccOutCurrent"
  Read CAN Message2/7 -> Bus Creator1/7  "CCURegenerateMode"
  Read CAN Message2/3 -> Bus Creator1/3  "CCUDccOutVoltage"
  Bus Creator/1 -> Subsystem/1(In1)
  Subsystem/2(MsgAvailable) -> MsgAvailable/1
  Read CAN Message2/1 -> Bus Creator1/1
  Read CAN Message2/6 -> Bus Creator1/6  "CCUControlMode"
  Read CAN Message3/5 -> Bus Creator3/5  "CCUInductor3Curr"
  Read CAN Message2/9 -> Bus Creator1/9  "CCUUnderBattVolt"
  Read CAN Message2/10 -> Bus Creator1/10  "CCUOverBattVolt"
  Read CAN Message2/11 -> Bus Creator1/11  "CCUOverInd1Curr"
  Read CAN Message2/12 -> Bus Creator1/12  "CCUOverInd2Curr"
  Read CAN Message2/13 -> Bus Creator1/13  "CCUOverInd3Curr"
  Read CAN Message2/14 -> Bus Creator1/14  "CCULeg1Failure"
  Read CAN Message2/15 -> Bus Creator1/15  "CCULeg2Failure"
  Read CAN Message2/16 -> Bus Creator1/16  "CCULeg3Failure"
  Read CAN Message2/17 -> Bus Creator1/17  "CCUOverOutVolt"

== system VHF_central_unit/ASW_ReadCAN/Read GeneratorSystem messages ==
  function : TriggerPort  TriggerType=function-call  VariantControl=(inherit)
  Bus Creator : BusCreator  Inputs=2
  Bus Creator1 : BusCreator  Inputs=17
  Bus Creator3 : BusCreator  Inputs=5
  Read CAN Message2 : SF_CanService_Libs/Read CAN Message  typeCAN=Connected  channel=CAN_A  mEn=off  msgInfo=VHF_VCU_Msg  msgItermStore=SCG_Status_VCU  msgIterm=SCG_Status_VCU  valid=on  stale=on  motoBit=off  setSignalName=on  flgCustomMonitorVariableRules=off  defineSignalName=on  prefixSignal='GenSys'  flgValTest=off  flgNoFixed=on  flgInheritForNoFixed=off  tSample=Task_Inherit  modeCode=Parameterless
  Read CAN Message3 : SF_CanService_Libs/Read CAN Message  typeCAN=Connected  channel=CAN_A  mEn=off  msgInfo=VHF_VCU_Msg  msgItermStore=SCG_ICE_Status  msgIterm=SCG_ICE_Status  valid=on  stale=on  motoBit=off  setSignalName=on  flgCustomMonitorVariableRules=off  defineSignalName=on  prefixSignal='GenSys'  flgValTest=off  flgNoFixed=on  flgInheritForNoFixed=off  tSample=Task_Inherit  modeCode=Parameterless
  Subsystem : Subsystem
  SCGmsgs : Outport
  MsgAvailable : Outport  Port=2
  MsgCount : Outport  Port=3
  wires:
  Read CAN Message2/15 -> Bus Creator1/15  "GenSysLeg1Failure"
  Subsystem/2(MsgAvailable) -> MsgAvailable/1
  Read CAN Message2/12 -> Bus Creator1/12  "GenSysOverInd1Curr"
  Read CAN Message2/13 -> Bus Creator1/13  "GenSysOverInd2Curr"
  Read CAN Message2/16 -> Bus Creator1/16  "GenSysLeg2Failure"
  Read CAN Message2/11 -> Bus Creator1/11  "GenSysOverOutVolt"
  Read CAN Message2/9 -> Bus Creator1/9  "GenSysLinkPosRelay"
  Read CAN Message2/7 -> Bus Creator1/7  "GenSysControlMode"
  Bus Creator1/1 -> Bus Creator/1  "SCG_Status_VCU"
  Read CAN Message2/10 -> Bus Creator1/10  "GenSysFaultControl"
  Read CAN Message3/5 -> Bus Creator3/5  "GenSysThrottle"
  Subsystem/3(MsgCount) -> MsgCount/1
  Read CAN Message2/17 -> Bus Creator1/17  "GenSysLeg3Failure"
  Read CAN Message3/2 -> Bus Creator3/2
  Subsystem/1(SCGmsgs) -> SCGmsgs/1
  Read CAN Message3/1 -> Bus Creator3/1
  Read CAN Message3/4 -> Bus Creator3/4  "GenSysMotorSpeed"
  Read CAN Message3/3 -> Bus Creator3/3  "GenSysMotorTorque"
  Bus Creator3/1 -> Bus Creator/2  "SCG_ICE_Status"
  Bus Creator/1 -> Subsystem/1(In1)
  Read CAN Message2/8 -> Bus Creator1/8  "GenSysAcRelayStatus"
  Read CAN Message2/14 -> Bus Creator1/14  "GenSysOverInd3Curr"
  Read CAN Message2/6 -> Bus Creator1/6  "GenSysGenCurrent"
  Read CAN Message2/5 -> Bus Creator1/5  "GenSysGenVoltage"
  Read CAN Message2/4 -> Bus Creator1/4  "GenSysDccOutCurrent"
  Read CAN Message2/3 -> Bus Creator1/3  "GenSysDccOutVoltage"
  Read CAN Message2/2 -> Bus Creator1/2
  Read CAN Message2/1 -> Bus Creator1/1

== system VHF_central_unit/ASW_ReadCAN/Read Motor1 messages ==
  function : TriggerPort  TriggerType=function-call  VariantControl=(inherit)
  Bus Creator : BusCreator  Inputs=2
  Bus Creator1 : BusCreator  Inputs=8
  Bus Creator3 : BusCreator  Inputs=4
  Read CAN Message2 : SF_CanService_Libs/Read CAN Message  typeCAN=Connected  channel=CAN_A  mEn=off  msgInfo=VHF_VCU_Msg  msgItermStore=Motor1_RUN_STATUS  msgIterm=Motor1_RUN_STATUS  valid=on  stale=on  motoBit=off  setSignalName=on  flgCustomMonitorVariableRules=off  defineSignalName=on  prefixSignal='Motor1'  flgValTest=off  flgNoFixed=on  flgInheritForNoFixed=off  tSample=Task_Inherit  modeCode=Parameterless
  Read CAN Message3 : SF_CanService_Libs/Read CAN Message  typeCAN=Connected  channel=CAN_A  mEn=off  msgInfo=VHF_VCU_Msg  msgItermStore=Motor1_ELEC_STATUS  msgIterm=Motor1_ELEC_STATUS  valid=on  stale=on  motoBit=off  setSignalName=on  flgCustomMonitorVariableRules=off  defineSignalName=on  prefixSignal='Motor1'  flgValTest=off  flgNoFixed=on  flgInheritForNoFixed=off  tSample=Task_Inherit  modeCode=Parameterless
  Subsystem : Subsystem
  Motor1msgs : Outport
  MsgAvailable : Outport  Port=2
  MsgCount : Outport  Port=3
  wires:
  Subsystem/2(MsgAvailable) -> MsgAvailable/1
  Subsystem/3(MsgCount) -> MsgCount/1
  Read CAN Message2/1 -> Bus Creator1/1
  Read CAN Message2/6 -> Bus Creator1/6  "Motor1Fault_Code"
  Read CAN Message2/3 -> Bus Creator1/3  "Motor1Run_direction"
  Subsystem/1(Motor1msgs) -> Motor1msgs/1
  Read CAN Message3/4 -> Bus Creator3/4  "Motor1DC_LinkCurrent"
  Bus Creator/1 -> Subsystem/1(In1)
  Read CAN Message2/5 -> Bus Creator1/5  "Motor1Motor_Speed"
  Read CAN Message3/3 -> Bus Creator3/3  "Motor1DC_LinkVoltage"
  Read CAN Message3/2 -> Bus Creator3/2
  Read CAN Message2/7 -> Bus Creator1/7  "Motor1ConsumptionMode"
  Bus Creator3/1 -> Bus Creator/2  "Motor1_ELEC_STATUS"
  Read CAN Message2/2 -> Bus Creator1/2
  Read CAN Message3/1 -> Bus Creator3/1
  Read CAN Message2/4 -> Bus Creator1/4  "Motor1Running_mode"
  Bus Creator1/1 -> Bus Creator/1  "Motor1_RUN_STATUS"
  Read CAN Message2/8 -> Bus Creator1/8  "Motor1SubtotalMileage"

== system VHF_central_unit/ASW_ReadCAN/Read Motor2 messages ==
  function : TriggerPort  TriggerType=function-call  VariantControl=(inherit)
  Bus Creator : BusCreator  Inputs=2
  Bus Creator1 : BusCreator  Inputs=8
  Bus Creator3 : BusCreator  Inputs=4
  Read CAN Message2 : SF_CanService_Libs/Read CAN Message  typeCAN=Connected  channel=CAN_A  mEn=off  msgInfo=VHF_VCU_Msg  msgItermStore=Motor2_RUN_STATUS  msgIterm=Motor2_RUN_STATUS  valid=on  stale=on  motoBit=off  setSignalName=on  flgCustomMonitorVariableRules=off  defineSignalName=on  prefixSignal='Motor2'  flgValTest=off  flgNoFixed=on  flgInheritForNoFixed=off  tSample=Task_Inherit  modeCode=Parameterless
  Read CAN Message3 : SF_CanService_Libs/Read CAN Message  typeCAN=Connected  channel=CAN_A  mEn=off  msgInfo=VHF_VCU_Msg  msgItermStore=Motor2_ELEC_STATUS  msgIterm=Motor2_ELEC_STATUS  valid=on  stale=on  motoBit=off  setSignalName=on  flgCustomMonitorVariableRules=off  defineSignalName=on  prefixSignal='Motor2'  flgValTest=off  flgNoFixed=on  flgInheritForNoFixed=off  tSample=Task_Inherit  modeCode=Parameterless
  Subsystem : Subsystem
  Motor2msgs : Outport
  MsgAvailable : Outport  Port=2
  MsgCount : Outport  Port=3
  wires:
  Subsystem/2(MsgAvailable) -> MsgAvailable/1
  Subsystem/3(MsgCount) -> MsgCount/1
  Read CAN Message2/1 -> Bus Creator1/1
  Read CAN Message2/6 -> Bus Creator1/6  "Motor2Fault_Code"
  Read CAN Message2/3 -> Bus Creator1/3  "Motor2Run_direction"
  Subsystem/1(Motor2msgs) -> Motor2msgs/1
  Read CAN Message3/4 -> Bus Creator3/4  "Motor2DC_LinkCurrent"
  Bus Creator/1 -> Subsystem/1(In1)
  Read CAN Message2/5 -> Bus Creator1/5  "Motor2Motor_Speed"
  Read CAN Message3/3 -> Bus Creator3/3  "Motor2DC_LinkVoltage"
  Read CAN Message3/2 -> Bus Creator3/2
  Read CAN Message2/7 -> Bus Creator1/7  "Motor2ConsumptionMode"
  Bus Creator3/1 -> Bus Creator/2  "Motor2_ELEC_STATUS"
  Read CAN Message2/2 -> Bus Creator1/2
  Read CAN Message3/1 -> Bus Creator3/1
  Read CAN Message2/4 -> Bus Creator1/4  "Motor2Running_mode"
  Bus Creator1/1 -> Bus Creator/1  "Motor2_RUN_STATUS"
  Read CAN Message2/8 -> Bus Creator1/8  "Motor2SubtotalMileage"

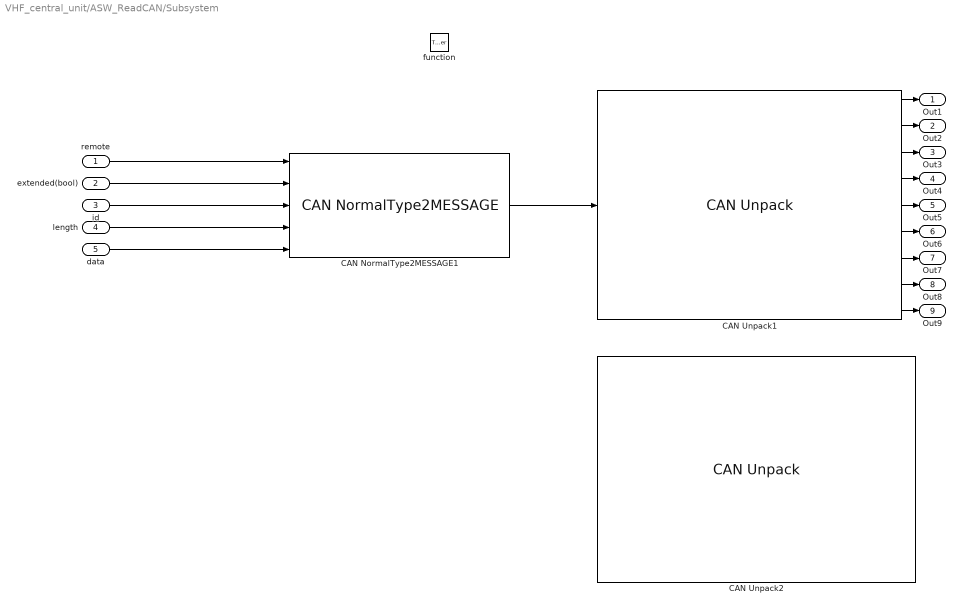
== system VHF_central_unit/ASW_ReadCAN/Subsystem ==
  remote : Inport
  extended(bool) : Inport  Port=2
  id : Inport  Port=3
  length : Inport  Port=4
  data : Inport  Port=5
  function : TriggerPort  TriggerType=function-call  VariantControl=(inherit)
  CAN NormalType2MESSAGE1 : CoderSF_BSW_Libs/CAN/CAN NormalType2MESSAGE
  CAN Unpack1 : canmsglib/CAN Unpack  CANdbFile=E:\Henrique\Poli\Pos-Mestrado2025\VCU HiL\VHF_Central_Unit\asw_libs\VHF_VCU_CAN.dbc  MsgList=BMS_CellVoltage1to8  MsgName=BMS_CellVoltage1to8  MsgIDType=Standard (11-bit identifier)  MsgIdentifier=805  MsgLength=8  SignalInfo={ 'CellVoltage1', '0', '8', 'LE', 'unsigned', 'Standard', '0', '0.02', '0', '0', '4.5'; 'CellVoltage2', '8', '8', 'LE', 'unsigned', 'Standard', '0', '0.02', '0', '0', '4.5'; 'CellVoltage3', '16', '8', 'LE', 'unsigned', 'Standard', '0', '0.02', '0', '0', '4.5'; 'CellVoltage4', '24', '8', 'LE', 'unsigned', 'Standard', '0', '0.02', '0', '0', '4.5'; 'CellVoltage5', '32', '8', 'LE', 'unsigned', 'Standard', '0', '0.02', '0', '0', '4.5'; 'CellVoltage6', '40', '8', 'LE', 'unsigned', 'Standard', '0', '0.02', '0', '0', '4.5'; 'CellVoltage7', '48', '8', 'LE', 'unsigned', 'Standard', '0', '0.02', '0', '0', '4.5'; 'CellVoltage8', '56', '8', 'LE', 'unsigned', 'Standard', '0', '0.02', '0', '0', '4.5' }  IDPort=off  TimestampPort=off  ErrorPort=on  RemotePort=off  LengthPort=off  StatusPort=off  ApplyMinMax=off
      settings: LibrarySourceBlock=embeddedtargetslib/Host Communication/CAN Unpack  DataFormat=CANdb specified signals
  CAN Unpack2 : canmsglib/CAN Unpack  CANdbFile=E:\Henrique\Poli\Pos-Mestrado2025\VCU HiL\VHF_Central_Unit\asw_libs\VHF_VCU_CAN.dbc  MsgList=BMS_CellVoltage9to16  MsgName=BMS_CellVoltage9to16  MsgIDType=Standard (11-bit identifier)  MsgIdentifier=806  MsgLength=8  SignalInfo={ 'CellVoltage10', '8', '8', 'LE', 'unsigned', 'Standard', '0', '0.02', '0', '0', '4.5'; 'CellVoltage11', '16', '8', 'LE', 'unsigned', 'Standard', '0', '0.02', '0', '0', '4.5'; 'CellVoltage12', '24', '8', 'LE', 'unsigned', 'Standard', '0', '0.02', '0', '0', '4.5'; 'CellVoltage13', '32', '8', 'LE', 'unsigned', 'Standard', '0', '0.02', '0', '0', '4.5'; 'CellVoltage14', '40', '8', 'LE', 'unsigned', 'Standard', '0', '0.02', '0', '0', '4.5'; 'CellVoltage15', '48', '8', 'LE', 'unsigned', 'Standard', '0', '0.02', '0', '0', '4.5'; 'CellVoltage16', '56', '8', 'LE', 'unsigned', 'Standard', '0', '0.02', '0', '0', '4.5'; 'CellVoltage9', '0', '8', 'LE', 'unsigned', 'Standard', '0', '0.02', '0', '0', '4.5' }  IDPort=off  TimestampPort=off  ErrorPort=on  RemotePort=off  LengthPort=off  StatusPort=off  ApplyMinMax=off
      settings: LibrarySourceBlock=embeddedtargetslib/Host Communication/CAN Unpack  DataFormat=CANdb specified signals
  Out1 : Outport
  Out2 : Outport  Port=2
  Out3 : Outport  Port=3
  Out4 : Outport  Port=4
  Out5 : Outport  Port=5
  Out6 : Outport  Port=6
  Out7 : Outport  Port=7
  Out8 : Outport  Port=8
  Out9 : Outport  Port=9
  wires:
  CAN Unpack1/9 -> Out9/1
  CAN NormalType2MESSAGE1/1 -> CAN Unpack1/1
  remote/1 -> CAN NormalType2MESSAGE1/1
  CAN Unpack1/8 -> Out8/1
  data/1 -> CAN NormalType2MESSAGE1/5
  extended(bool)/1 -> CAN NormalType2MESSAGE1/2
  length/1 -> CAN NormalType2MESSAGE1/4
  id/1 -> CAN NormalType2MESSAGE1/3
  CAN Unpack1/6 -> Out6/1
  CAN Unpack1/5 -> Out5/1
  CAN Unpack1/1 -> Out1/1
  CAN Unpack1/4 -> Out4/1
  CAN Unpack1/2 -> Out2/1
  CAN Unpack1/3 -> Out3/1
  CAN Unpack1/7 -> Out7/1

== system VHF_central_unit/ASW_ReadCAN/Subsystem1 ==
  remote : Inport
  extended(bool) : Inport  Port=2
  id : Inport  Port=3
  length : Inport  Port=4
  data : Inport  Port=5
  function : TriggerPort  TriggerType=function-call  VariantControl=(inherit)
  CAN NormalType2MESSAGE1 : CoderSF_BSW_Libs/CAN/CAN NormalType2MESSAGE
  CAN Unpack1 : canmsglib/CAN Unpack  CANdbFile=E:\Henrique\Poli\Pos-Mestrado2025\VCU HiL\VHF_Central_Unit\asw_libs\VHF_VCU_CAN.dbc  MsgList=VCUCommands  MsgName=VCUCommands  MsgIDType=Standard (11-bit identifier)  MsgIdentifier=16  MsgLength=8  SignalInfo={'LinkVoltageTarget','8','8','LE','unsigned','Standard','0','0.2','70','70','120';'SpeedICE','16','16','LE','unsigned','Standard','0','1','0','-Inf','Inf';'ThrottleTarget','0','8','LE','unsigned','Standard','0','0.5','0','0','100'}  IDPort=off  TimestampPort=off  ErrorPort=off  RemotePort=off  LengthPort=off  StatusPort=on  ApplyMinMax=off
      settings: LibrarySourceBlock=embeddedtargetslib/Host Communication/CAN Unpack  DataFormat=CANdb specified signals
  Out1 : Outport
  Out2 : Outport  Port=2
  Out3 : Outport  Port=3
  Out4 : Outport  Port=4
  wires:
  CAN NormalType2MESSAGE1/1 -> CAN Unpack1/1
  remote/1 -> CAN NormalType2MESSAGE1/1
  data/1 -> CAN NormalType2MESSAGE1/5
  extended(bool)/1 -> CAN NormalType2MESSAGE1/2
  length/1 -> CAN NormalType2MESSAGE1/4
  id/1 -> CAN NormalType2MESSAGE1/3
  CAN Unpack1/1 -> Out1/1
  CAN Unpack1/4 -> Out4/1
  CAN Unpack1/2 -> Out2/1
  CAN Unpack1/3 -> Out3/1

== system VHF_central_unit/ASW_SensorInputs/02 vehicle motion request ==
  sigInDrvPedacc_pct : Inport
  01 driver torque demand : Subsystem
  Task_Call2 : CoderSF_BSW_Libs/Task Scheduler/Task Trigger  tasktimeIndex=Task_L20ms
  vehDrv_trqReq : Outport
  wires:
  Task_Call2/1 -> 01 driver torque demand/Trigger
  01 driver torque demand/1(vehDrv_trqReq1) -> vehDrv_trqReq/1
  sigInDrvPedacc_pct/1 -> 01 driver torque demand/1(sigInDrvPedacc_pct1)

== system VHF_central_unit/ASW_SensorInputs/Accelerator read ==
  Accelerator In : Subsystem
  Task Trigger : CoderSF_BSW_Libs/Task Scheduler/Task Trigger  tasktimeIndex=Task_H20ms
  thrtl : Outport
  wires:
  Task Trigger/1 -> Accelerator In/Trigger
  Accelerator In/1(thrtl) -> thrtl/1

== system VHF_central_unit/ASW_SensorInputs/Brake read ==
  Get Brake signal : Subsystem
  Task Trigger : CoderSF_BSW_Libs/Task Scheduler/Task Trigger  tasktimeIndex=Task_L20ms
  brk : Outport
  wires:
  Task Trigger/1 -> Get Brake signal/Trigger
  Get Brake signal/1(brk) -> brk/1

== system VHF_central_unit/ASW_SensorInputs/MEMS sensor read ==
  Estimate speed : Subsystem
  Read Sensor Data : Subsystem
  Task Trigger1 : CoderSF_BSW_Libs/Task Scheduler/Task Trigger  Priority=2  tasktimeIndex=Task_L50ms  PrioritySet=2
  Task Trigger4 : CoderSF_BSW_Libs/Task Scheduler/Task Trigger  Priority=1  tasktimeIndex=Task_L50ms  PrioritySet=1
  ID : Outport
  V : Outport  Port=2
  Orientation : Outport  Port=3
  Gyro : Outport  Port=4
  Temp : Outport  Port=5
  wires:
  Task Trigger4/1 -> Read Sensor Data/Trigger
  Task Trigger1/1 -> Estimate speed/Trigger
  Read Sensor Data/3(Gyro) -> Gyro/1, Estimate speed/2(Gyro)
  Read Sensor Data/2(Accel) -> Estimate speed/1(Accel)
  Read Sensor Data/1(ID) -> ID/1
  Estimate speed/2(Orientation) -> Orientation/1
  Read Sensor Data/4(Temp) -> Temp/1
  Estimate speed/1(Vspeed) -> V/1

== system VHF_central_unit/ASW_SensorInputs/Output Routing ==
  In1 : Inport
  ToChassis : Outport
  ToPowertrain : Outport  Port=2
  wires:
  In1/1 -> ToChassis/1

== system VHF_central_unit/ASW_SensorInputs/Read BMS msgs ==
  Subsystem1 : Subsystem
  Task Trigger : CoderSF_BSW_Libs/Task Scheduler/Task Trigger  tasktimeIndex=Task_L20ms
  Out1 : Outport
  wires:
  Subsystem1/1(Out1) -> Out1/1
  Task Trigger/1 -> Subsystem1/Trigger

== system VHF_central_unit/ASW_SensorInputs/Read DCDC converter msgs ==
  Subsystem1 : Subsystem
  Task Trigger : CoderSF_BSW_Libs/Task Scheduler/Task Trigger  tasktimeIndex=Task_L20ms
  Out1 : Outport
  wires:
  Subsystem1/1(Out1) -> Out1/1
  Task Trigger/1 -> Subsystem1/Trigger

== system VHF_central_unit/ASW_SensorInputs/Read GenSys msgs ==
  Subsystem1 : Subsystem
  Task Trigger : CoderSF_BSW_Libs/Task Scheduler/Task Trigger  tasktimeIndex=Task_L20ms
  Out1 : Outport
  wires:
  Subsystem1/1(Out1) -> Out1/1
  Task Trigger/1 -> Subsystem1/Trigger

== system VHF_central_unit/ASW_SensorInputs/Read Inverter 1 ==
  Subsystem1 : Subsystem
  Task Trigger : CoderSF_BSW_Libs/Task Scheduler/Task Trigger  tasktimeIndex=Task_L20ms
  Out1 : Outport
  wires:
  Task Trigger/1 -> Subsystem1/Trigger
  Subsystem1/1(Out1) -> Out1/1

== system VHF_central_unit/ASW_SensorInputs/Read Inverter 2 ==
  Subsystem1 : Subsystem
  Task Trigger : CoderSF_BSW_Libs/Task Scheduler/Task Trigger  tasktimeIndex=Task_L20ms
  Out1 : Outport
  wires:
  Subsystem1/1(Out1) -> Out1/1
  Task Trigger/1 -> Subsystem1/Trigger
